simulink model "crane_model_mpc[1]"  (R2023a)
settings: Solver=ode45  StartTime=0.0  StopTime=10.0  RelTol=1e-3  EnableMultiTasking=on
settings Model: Creator=The MathWorks, Inc.  LastModifiedBy=ASUS
settings SolverCC: AlgebraicLoopSolver=TrustRegion  MinimalZcImpactIntegration=on  MaxZcPerStep=1
settings DataIOCC: LimitDataPoints=on  ReturnWorkspaceOutputs=off
settings OptimizationCC: LifeSpan=inf
settings DebuggingCC: UnconnectedInputMsg=warning  UnconnectedOutputMsg=warning  UnconnectedLineMsg=warning  AllowSymbolicDim=off  SFUnexpectedBacktrackingDiag=warning  SFNoUnconditionalDefaultTransitionDiag=warning  SFExecutionAtInitializationDiag=none  ArithmeticOperatorsInVariantConditions=warning
settings ModelReferenceCC: EnableRefExpFcnMdlSchedulingChecks=on  PropagateSignalLabelsOutOfModel=off
settings SFSimCC: SimUseLocalCustomCode=off  CustomCodeUndefinedFunction=UseInterfaceOnly
settings RTWCC: RTWUseLocalCustomCode=off
settings CodeAppCC: StateflowObjectComments=on
settings GRTTargetCC: TargetLangStandard=C89/C90 (ANSI)
settings ConfigComp: CovScope=ReferencedModels  CovMetricSettings=dw  CovSaveCumulativeToWorkspaceVar=on  CovSaveSingleToWorkspaceVar=on  CovExternalEMLEnable=off
settings SimscapeCC: SimscapeNormalizeSystem=off

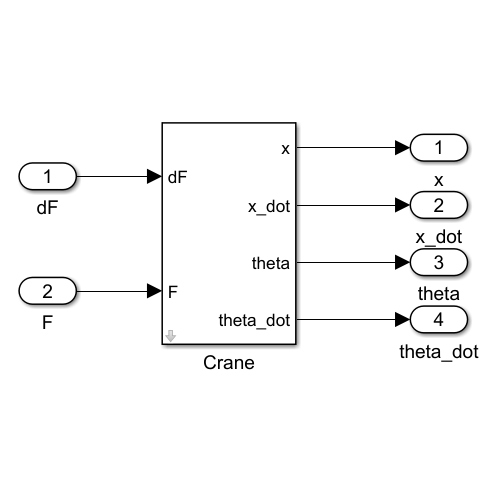
[thumbnail: Simulink's stored preview of the top-level diagram]
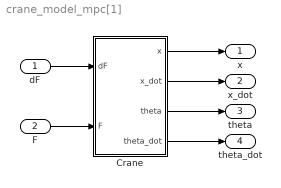
== system crane_model_mpc[1] ==
  dF : Inport
  F : Inport  Port=2
  Crane : Subsystem  mask{mCartPara=2, mPendPara=0.5, gPara=9.81, LPara=5, KdPara=0}
      mask prompts: mCartPara "Mass of Cart"; mPendPara "Mass of Pendulum"; gPara "Gravity"; LPara "Length of Pendulum"; KdPara "Friction coefficient of Cart"
      mask help: Pendulum and Cart System
      mask init:
      | mCart = str2double(get_param(gcb,'mCartPara'));
      | mPend = str2double(get_param(gcb,'mPendPara'));
      | g = str2double(get_param(gcb,'gPara'));
      | L = str2double(get_param(gcb,'LPara'));
      | Kd = str2double(get_param(gcb,'KdPara'));
  x : Outport  VectorParamsAs1DForOutWhenUnconnected=off
  x_dot : Outport  Port=2  VectorParamsAs1DForOutWhenUnconnected=off
  theta : Outport  Port=3  VectorParamsAs1DForOutWhenUnconnected=off
  theta_dot : Outport  Port=4  VectorParamsAs1DForOutWhenUnconnected=off
  wires:
  F/1 -> Crane/2(F)
  Crane/1(x) -> x/1
  Crane/4(theta_dot) -> theta_dot/1
  Crane/3(theta) -> theta/1
  Crane/2(x_dot) -> x_dot/1
  dF/1 -> Crane/1(dF)

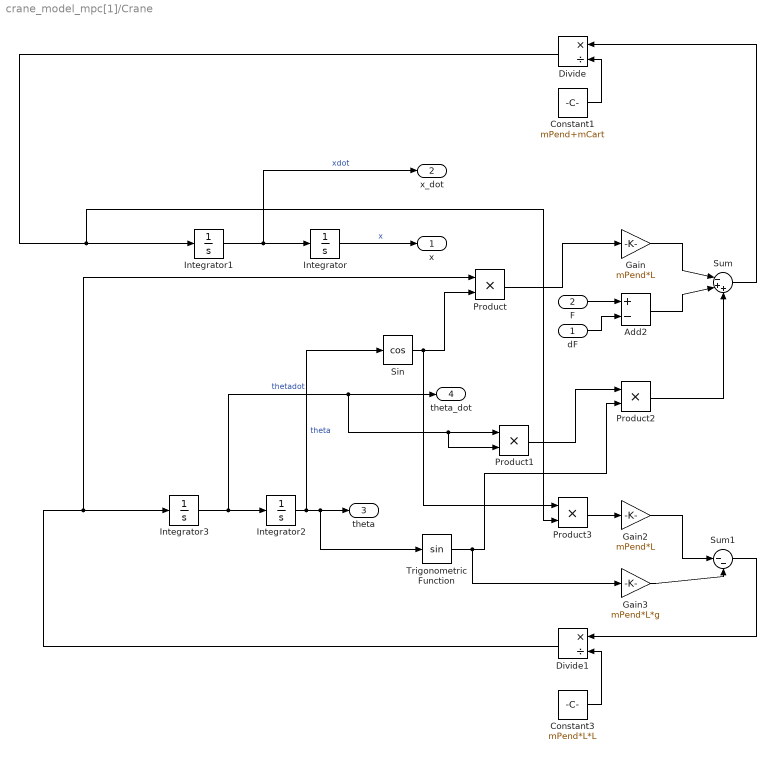
== system crane_model_mpc[1]/Crane ==
  dF : Inport
  F : Inport  Port=2
  Add2 : Sum  Inputs=+-
  Constant1 : Constant  Value=mPend+mCart
  Constant3 : Constant  Value=mPend*L*L
  Divide : Product  Inputs=*/
  Divide1 : Product  Inputs=*/
  Gain : Gain  Gain=mPend*L
  Gain2 : Gain  Gain=mPend*L
  Gain3 : Gain  Gain=mPend*L*g
  Integrator : Integrator  ContinuousStateAttributes='x'
  Integrator1 : Integrator  ContinuousStateAttributes='xdot'
  Integrator2 : Integrator  ContinuousStateAttributes='theta'
  Integrator3 : Integrator  ContinuousStateAttributes='thetadot'
  Product{,1..3} (4 alike) : Product
  Sin : Trigonometry  Operator=cos
  Sum : Sum  Inputs=|-++
  Sum1 : Sum  Inputs=|--
  Trigonometric Function : Trigonometry
  x : Outport  VectorParamsAs1DForOutWhenUnconnected=off
  x_dot : Outport  Port=2  VectorParamsAs1DForOutWhenUnconnected=off
  theta : Outport  Port=3  VectorParamsAs1DForOutWhenUnconnected=off
  theta_dot : Outport  Port=4  VectorParamsAs1DForOutWhenUnconnected=off
  wires:
  Product/1 -> Gain/1
  Divide/1 -> Product3/2, Integrator1/1
  Constant1/1 -> Divide/2
  Sum1/1 -> Divide1/1
  Gain2/1 -> Sum1/1
  Product2/1 -> Sum/3
  Gain/1 -> Sum/1
  Sin/1 -> Product3/1, Product/2
  Divide1/1 -> Product/1, Integrator3/1
  Product1/1 -> Product2/1
  F/1 -> Add2/1
  Add2/1 -> Sum/2
  dF/1 -> Add2/2
  Trigonometric Function/1 -> Gain3/1, Product2/2
  Product3/1 -> Gain2/1
  Integrator3/1 -> Integrator2/1, Product1/2, Product1/1, theta_dot/1  "thetadot"
  Sum/1 -> Divide/1
  Integrator2/1 -> Sin/1, Trigonometric Function/1, theta/1  "theta"
  Constant3/1 -> Divide1/2
  Integrator1/1 -> x_dot/1, Integrator/1  "xdot"
  Gain3/1 -> Sum1/2
  Integrator/1 -> x/1  "x"
